simulink model "Vehicle_Dynamics"  (R2024b)
settings: Solver=FixedStepAuto  StartTime=0.0  StopTime=10.0  RelTol=1e-3
values from neighbouring files (symbols this model uses):
  A_front = 0.5    [init_params.m]
  Cd = 0.35    [init_params.m]
  eff_drive = 0.95    [init_params.m]
  f_roll = 0.015    [init_params.m]
  g = g_to_ms2    (= 9.81)    [init_params.m]
  ig = 5.0    (= 5)    [init_params.m]
  Jm = 0.25    [init_params.m]
  Jw = 4.0    (= 4)    [init_params.m]
  m = 1500    [init_params.m]
  max_brake_torque = 1500 * 4    (= 6000)    [init_params.m]
  rho_air = 1.226    [init_params.m]
  rw = 0.28    [init_params.m]
  v_ego_init = 50 * kmh_to_ms    (= 13.8888888889)    [init_params.m]
  x_ego_init = 0    [init_params.m]
settings Model: Creator=ezers  LastModifiedBy=ezers
settings DataIOCC: ExternalInput=ds  LoadExternalInput=on

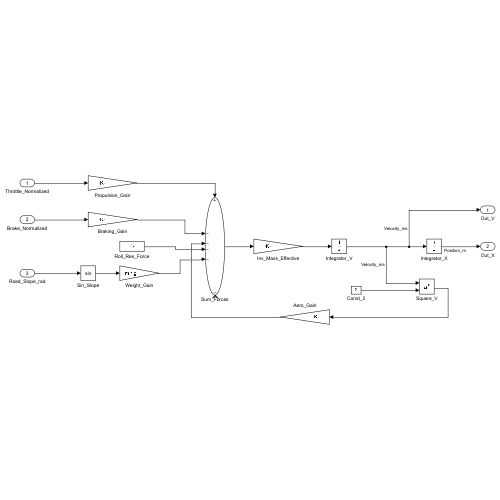
[thumbnail: Simulink's stored preview of the top-level diagram]
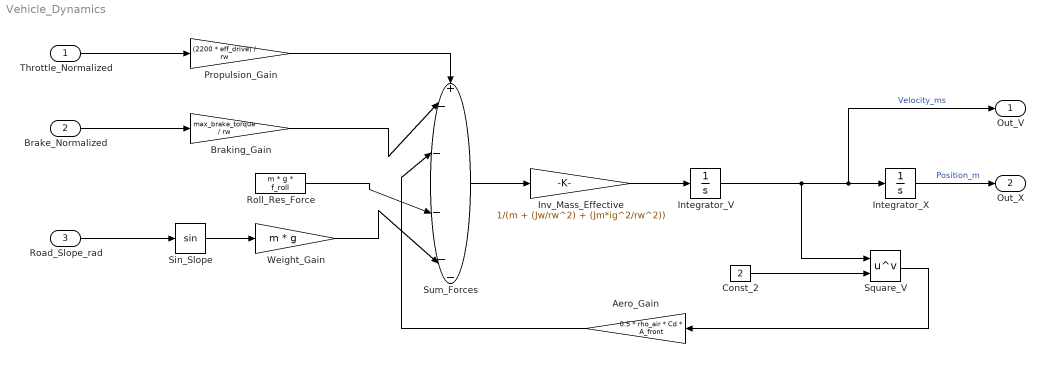
== system Vehicle_Dynamics ==
  Throttle_Normalized : Inport
  Brake_Normalized : Inport  Port=2
  Road_Slope_rad : Inport  Port=3
  Aero_Gain : Gain  Gain=0.5 * rho_air * Cd * A_front
  Braking_Gain : Gain  Gain=max_brake_torque / rw
  Const_2 : Constant  Value=2
  Integrator_V : Integrator  InitialCondition=v_ego_init
  Integrator_X : Integrator  InitialCondition=x_ego_init
  Inv_Mass_Effective : Gain  Gain=1/(m + (Jw/rw^2) + (Jm*ig^2/rw^2))
  Propulsion_Gain : Gain  Gain=(2200 * eff_drive) / rw
  Roll_Res_Force : Constant  Value=m * g * f_roll
  Sin_Slope : Trigonometry
  Square_V : Math  Operator=pow
  Sum_Forces : Sum  Inputs=+-----
  Weight_Gain : Gain  Gain=m * g
  Out_V : Outport
  Out_X : Outport  Port=2
  wires:
  Throttle_Normalized/1 -> Propulsion_Gain/1
  Brake_Normalized/1 -> Braking_Gain/1
  Propulsion_Gain/1 -> Sum_Forces/1
  Braking_Gain/1 -> Sum_Forces/2
  Roll_Res_Force/1 -> Sum_Forces/4
  Road_Slope_rad/1 -> Sin_Slope/1
  Sin_Slope/1 -> Weight_Gain/1
  Weight_Gain/1 -> Sum_Forces/5
  Sum_Forces/1 -> Inv_Mass_Effective/1
  Inv_Mass_Effective/1 -> Integrator_V/1
  Integrator_V/1 -> Out_V/1, Integrator_X/1, Square_V/1  "Velocity_ms"
  Const_2/1 -> Square_V/2
  Square_V/1 -> Aero_Gain/1
  Aero_Gain/1 -> Sum_Forces/3
  Integrator_X/1 -> Out_X/1  "Position_m"
